simulink model "TestingModelWithSimpleNoise"  (R2021a)
settings: Solver=VariableStepAuto  StartTime=0.0  StopTime=0.1  RelTol=1e-3
values from neighbouring files (symbols this model uses):
  attn_atm = 1.18    [PrepareLink.m]
  attn_rain = 0    [PrepareLink.m]
  bitRate = 5e6    (= 5000000)    [PrepareLink.m]
  bitsPerFrame = 32    [PrepareLink.m]
  G_ant_rx = 42.8    [PrepareLink.m]
  G_ant_tx = 25    [PrepareLink.m]
  G_bpf_rx = 10^(-0.6/10)    (= 0.870963589956)    [PrepareLink.m]
  G_bpf_rx2 = 10^(-0.6/10)    (= 0.870963589956)    [PrepareLink.m]
  G_hpa_rx = 10^(20/10)    (= 100)    [PrepareLink.m]
  G_hpa_rx2 = 10^(35/10)    (= 3162.27766017)    [PrepareLink.m]
  G_lna_rx = 10^(10/10)    (= 10)    [PrepareLink.m]
  G_lpf_rx = 10^(-1.6/10)    (= 0.691830970919)    [PrepareLink.m]
  G_mix2_rx = 10^(-8/10)    (= 0.158489319246)    [PrepareLink.m]
  G_mix_rx = 10^(-8/10)    (= 0.158489319246)    [PrepareLink.m]
  maxDoppler = 650e3    (= 650000)    [PrepareLink.m]
undefined symbols (not defined in the file or in its folder): doppler, FSPL_TX, pskmod
libraries: commrflib2 x10, commfilt2 x3, commrfcorlib x2, commdigbbndpm3 x2, commcnvcod2 x2, commutil2 x2, commrandsrc3 x1, commsync2 x1, commsink2 x1, commchan3 x1
settings Model: Creator=drewd  LastModifiedBy=drewd

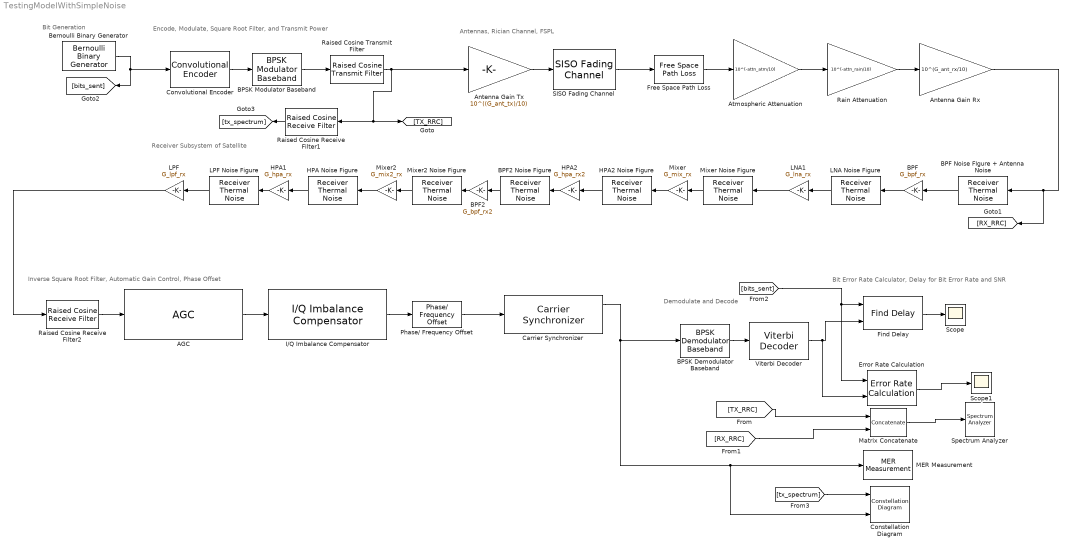
== system TestingModelWithSimpleNoise ==
  note: Bit Generation
  note: Demodulate and Decode
  note: Bit Error Rate Calculator, Delay for Bit Error Rate and SNR
  note: Inverse Square Root Filter, Automatic Gain Control, Phase Offset
  note: Receiver Subsystem of Satellite
  note: Encode, Modulate, Square Root Filter, and Transmit Power
  note: Antennas, Rician Channel, FSPL
  AGC : commrfcorlib/AGC  LegacyMode=off  DetectorMethod=Rectifier  LoopMethod=Linear  UpdatePeriod=100  StepSize=0.1  AdaptationStepSize=0.01  DesiredOutputPower=1  AveragingLength=256  MaximumGain=30  MaxPowerGain=60  GainOutputPort=off  InputPowerOutputPort=off  SimulateUsing=Interpreted execution
  Antenna Gain Rx : Gain  Gain=10^(G_ant_rx/10)
  Antenna Gain Tx : Gain  Gain=10^((G_ant_tx)/10)
  Atmospheric Attenuation : Gain  Gain=10^(-attn_atm/10)
  BPF : Gain  Gain=G_bpf_rx
  BPF Noise FIgure + Antenna Noise : commrflib2/Receiver Thermal Noise  method=Noise figure  ntemp=290  nfigure=0.6  nfactor=2  add290KAntennaNoise=on  seed=67987
      settings: SourceProductBaseCode=CM
  BPF2 : Gain  Gain=G_bpf_rx2
  BPF2 Noise Figure : commrflib2/Receiver Thermal Noise  method=Noise figure  ntemp=290  nfigure=8  nfactor=2  add290KAntennaNoise=off  seed=67987
      settings: SourceProductBaseCode=CM
  BPSK Demodulator Baseband : commdigbbndpm3/BPSK Demodulator Baseband  DecType=Hard decision  VarSource=Dialog  Variance=1  Ph=0  outDtype=Inherit via internal rule  derotateFactorWordLen=16  derotateFactorDataTypeStr=Inherit: Same word length as input  derotateFactorLastDataTypeStr=Inherit: Same word length as input
  BPSK Modulator Baseband : commdigbbndpm3/BPSK Modulator Baseband  Ph=0  outDtype=double  outWordLen=16  outUDDataType=sfix(16)  outFracLenMode=Best precision  outFracLen=15  outDataTypeStr=double  outLastDataTypeStr=double
  Bernoulli Binary Generator : commrandsrc3/Bernoulli Binary Generator  ProbabilityOfZero=0.5  SeedSource=Auto  Seed=0  SampleTime=1/bitRate  SamplesPerFrame=bitsPerFrame  OutputDataType=double  SimulateUsing=Interpreted execution
  Carrier Synchronizer : commsync2/Carrier Synchronizer  Modulation=BPSK  ModulationPhaseOffset=Auto  CustomPhaseOffset=0  SamplesPerSymbol=2  DampingFactor=0.707  NormalizedLoopBandwidth=0.01  EstimatedPhaseErrorOutputPort=on  SimulateUsing=Code generation
  Constellation Diagram : ConstellationDiagram  NumInputPorts=2
  Convolutional Encoder : commcnvcod2/Convolutional Encoder  trellis=poly2trellis([5,4], [23 35 0; 0 5 13])  opMode=Continuous  DelayedResetAction=on  hasIniStPort=off  hasFinStPort=off  usePuncVector=off  punctureVector=[1; 1; 0; 1; 0; 1]  reset=Unused parameter value
      settings: SourceProductBaseCode=CM
  Error Rate Calculation : commsink2/Error Rate Calculation  N=72  st_delay=0  cp_mode=Entire frame  subframe=[]  PMode=Port  WsName=ErrorVec  RsMode2=off  stop=off  numErr=100  maxBits=1e6
  Find Delay : commutil2/Find Delay  corrLength=5000  chgSigOP=off  stopUpdate=off  numConstDelay=3
      settings: SourceProductBaseCode=CM
  Free Space Path Loss : commrflib2/Free Space Path Loss  mode=Distance and Frequency  dB=-FSPL_TX  d=R  fc=fc_tx
      settings: SourceProductBaseCode=CM
  HPA Noise Figure : commrflib2/Receiver Thermal Noise  method=Noise figure  ntemp=290  nfigure=4  nfactor=2  add290KAntennaNoise=off  seed=67987
      settings: SourceProductBaseCode=CM
  HPA1 : Gain  Gain=G_hpa_rx
  HPA2 : Gain  Gain=G_hpa_rx2
  HPA2 Noise Figure : commrflib2/Receiver Thermal Noise  method=Noise figure  ntemp=290  nfigure=7.0  nfactor=2  add290KAntennaNoise=off  seed=67987
      settings: SourceProductBaseCode=CM
  I/Q Imbalance Compensator : commrfcorlib/I//Q Imbalance Compensator  CoefficientSource=Estimated from input signal  InitialCoefficient=0 + 0j  StepSizeSource=Property  StepSize=0.00001  AdaptInputPort=off  CoefficientOutputPort=off  SimulateUsing=Code generation
      settings: SourceProductBaseCode=CM
  LNA Noise Figure : commrflib2/Receiver Thermal Noise  method=Noise figure  ntemp=290  nfigure=5  nfactor=2  add290KAntennaNoise=off  seed=67987
      settings: SourceProductBaseCode=CM
  LNA1 : Gain  Gain=G_lna_rx
  LPF : Gain  Gain=G_lpf_rx
  LPF Noise Figure : commrflib2/Receiver Thermal Noise  method=Noise figure  ntemp=290  nfigure=1.6  nfactor=2  add290KAntennaNoise=off  seed=67987
      settings: SourceProductBaseCode=CM
  MER Measurement : commutil2/MER Measurement  ReferenceSignalSource=Estimated from reference constellation  ReferenceConstellation=pskmod(0:1,2,0)  MeasurementIntervalSource=Entire history  MeasurementInterval=100  AveragingDimensions=1  MinimumMEROutputPort=off  XPercentileMEROutputPort=off  XPercentileValue=95  SymbolCountOutputPort=off  SimulateUsing=Interpreted execution
      settings: SourceProductBaseCode=CM
  Matrix Concatenate : Concatenate  Mode=Multidimensional array  ConcatenateDimension=2
  Mixer : Gain  Gain=G_mix_rx
  Mixer Noise Figure : commrflib2/Receiver Thermal Noise  method=Noise figure  ntemp=290  nfigure=20  nfactor=2  add290KAntennaNoise=off  seed=67987
      settings: SourceProductBaseCode=CM
  Mixer2 : Gain  Gain=G_mix2_rx
  Mixer2 Noise Figure : commrflib2/Receiver Thermal Noise  method=Noise figure  ntemp=290  nfigure=20  nfactor=2  add290KAntennaNoise=off  seed=67987
      settings: SourceProductBaseCode=CM
  Phase/ Frequency Offset : commrflib2/Phase// Frequency Offset  phaseOffset=90  freqPort=off  freqOffset=-maxDoppler
  Rain Attenuation : Gain  Gain=10^(-attn_rain/10)
  Raised Cosine Receive Filter1 : commfilt2/Raised Cosine Receive Filter  filtType=Square root  R=0.2  filtSpan=6  N=bitsPerFrame  downFactor=bitsPerFrame  downOffset=0  filterGain=1/sqrt(bitsPerFrame)  InputProcessing=Columns as channels (frame based)  RateOptions=Enforce single-rate processing  framing=Mute  checkCoeff=off  variableName=rcRxFilt1  currentFiltSpan=10  D=5  inputOffset=0  sampMode=Mute  saveAsFlag=0  rateMode=Downsampling  checkGain=Normalized  launchFVT=on  roundingMode=Floor  overflowMode=off  coeffDataTypeStr=Inherit: Same word length as input  coeffMin=[]  coeffMax=[]  coeffLastDataTypeStr=Inherit: Same word length as input  accumDataTypeStr=Inherit: Same as product output  accumLastDataTypeStr=Inherit: Same as product output  outputDataTypeStr=Inherit: Same as accumulator  outputMin=[]  outputMax=[]  outputLastDataTypeStr=Inherit: Same as accumulator
  Raised Cosine Receive Filter2 : commfilt2/Raised Cosine Receive Filter  filtType=Square root  R=0.2  filtSpan=6  N=bitsPerFrame  downFactor=bitsPerFrame  downOffset=0  filterGain=1/sqrt(bitsPerFrame)  InputProcessing=Columns as channels (frame based)  RateOptions=Enforce single-rate processing  framing=Mute  checkCoeff=off  variableName=rcRxFilt2  currentFiltSpan=10  D=5  inputOffset=0  sampMode=Mute  saveAsFlag=0  rateMode=Downsampling  checkGain=Normalized  launchFVT=on  roundingMode=Floor  overflowMode=off  coeffDataTypeStr=Inherit: Same word length as input  coeffMin=[]  coeffMax=[]  coeffLastDataTypeStr=Inherit: Same word length as input  accumDataTypeStr=Inherit: Same as product output  accumLastDataTypeStr=Inherit: Same as product output  outputDataTypeStr=Inherit: Same as accumulator  outputMin=[]  outputMax=[]  outputLastDataTypeStr=Inherit: Same as accumulator
  Raised Cosine Transmit Filter : commfilt2/Raised Cosine Transmit Filter  filtType=Square root  R=0.2  filtSpan=6  N=bitsPerFrame  filterGain=sqrt(bitsPerFrame)  InputProcessing=Columns as channels (frame based)  RateOptions=Enforce single-rate processing  framing=Mute  checkCoeff=off  variableName=rcTxFilt  checkGain=Normalized  sampMode=Mute  saveAsFlag=0  currentFiltSpan=10  D=(10)/2  launchFVT=on  roundingMode=Floor  overflowMode=off  coeffDataTypeStr=Inherit: Same word length as input  coeffMin=[]  coeffMax=[]  coeffLastDataTypeStr=Inherit: Same word length as input  outputDataTypeStr=Inherit: Same as accumulator  outputMin=[]  outputMax=[]  outputLastDataTypeStr=Inherit: Same as accumulator
  SISO Fading Channel : commchan3/SISO Fading Channel  InheritSampleRate=on  SampleRate=1  PathDelays=pathDelays  AveragePathGains=AverageGains  NormalizePathGains=on  FadingDistribution=Rician  KFactor=Kfactor  DirectPathDopplerShift=maxDoppler  DirectPathInitialPhase=0  MaximumDopplerShift=20  DopplerSpectrum=doppler('Jakes')  RandomStream=mt19937ar with seed  Seed=15  PathGainsOutputPort=off  ChannelFilterDelayOutputPort=off  SimulateUsing=Interpreted execution  Visualization=Doppler spectrum  PathsForDopplerDisplay=1  SamplesToDisplay=25%
  Scope : Scope
  Scope1 : Scope
  Spectrum Analyzer : SpectrumAnalyzer
  Viterbi Decoder : commcnvcod2/Viterbi Decoder  trellis=poly2trellis([5,4], [23 35 0; 0 5 13])  isPunctured=off  punctureVector=[1; 1; 0; 1; 0; 1]  erasures=off  dectype=Hard decision  nsdecb=4  runSigValErrCheck=off  tbdepth=34  opmode=Continuous  reset=off  delayedResetAction=on  smWordLength=16  outDataType=double
      settings: SourceProductBaseCode=CM
  wires:
  Antenna Gain Tx/1 -> SISO Fading Channel/1
  BPF Noise FIgure + Antenna Noise/1 -> BPF/1
  BPF/1 -> LNA Noise Figure/1
  HPA Noise Figure/1 -> HPA1/1
  LNA Noise Figure/1 -> LNA1/1
  LNA1/1 -> Mixer Noise Figure/1
  Mixer Noise Figure/1 -> Mixer/1
  LPF Noise Figure/1 -> LPF/1
  Error Rate Calculation/1 -> Scope1/1
  Convolutional Encoder/1 -> BPSK Modulator Baseband/1
  Atmospheric Attenuation/1 -> Rain Attenuation/1
  Rain Attenuation/1 -> Antenna Gain Rx/1
  Free Space Path Loss/1 -> Atmospheric Attenuation/1
  Antenna Gain Rx/1 -> BPF Noise FIgure + Antenna Noise/1, [RX_RRC]
  HPA1/1 -> LPF Noise Figure/1
  Mixer/1 -> HPA2 Noise Figure/1
  HPA2 Noise Figure/1 -> HPA2/1
  BPF2 Noise Figure/1 -> BPF2/1
  HPA2/1 -> BPF2 Noise Figure/1
  Mixer2 Noise Figure/1 -> Mixer2/1
  BPF2/1 -> Mixer2 Noise Figure/1
  Mixer2/1 -> HPA Noise Figure/1
  [TX_RRC] -> Matrix Concatenate/1
  Bernoulli Binary Generator/1 -> [bits_sent], Convolutional Encoder/1
  [bits_sent] -> Error Rate Calculation/1, Find Delay/1
  Find Delay/1 -> Scope/1
  BPSK Modulator Baseband/1 -> Raised Cosine Transmit Filter/1
  BPSK Demodulator Baseband/1 -> Viterbi Decoder/1
  Viterbi Decoder/1 -> Error Rate Calculation/2, Find Delay/2
  Raised Cosine Transmit Filter/1 -> Antenna Gain Tx/1, Raised Cosine Receive Filter1/1, [TX_RRC]
  LPF/1 -> Raised Cosine Receive Filter2/1
  AGC/1 -> I/Q Imbalance Compensator/1
  Raised Cosine Receive Filter2/1 -> AGC/1
  SISO Fading Channel/1 -> Free Space Path Loss/1
  I/Q Imbalance Compensator/1 -> Phase/ Frequency Offset/1
  [RX_RRC] -> Matrix Concatenate/2
  Matrix Concatenate/1 -> Spectrum Analyzer/1
  Carrier Synchronizer/1 -> Constellation Diagram/2, MER Measurement/1, BPSK Demodulator Baseband/1
  Phase/ Frequency Offset/1 -> Carrier Synchronizer/1
  Raised Cosine Receive Filter1/1 -> [tx_spectrum]
  [tx_spectrum] -> Constellation Diagram/1
